simulink model "step3"  (R2021a)
settings: Solver=VariableStepAuto  StartTime=0.0  StopTime=100.0  RelTol=1e-3
settings Model: Creator=konsta  LastModifiedBy=konsta

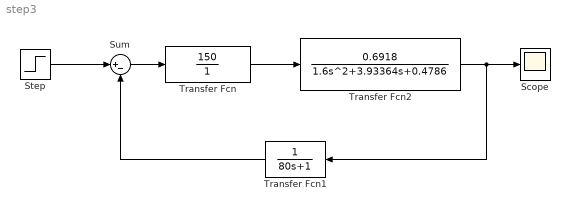
== system step3 ==
  Scope : Scope
  Step : Step  SampleTime=0
  Sum : Sum  Inputs=|+-
  Transfer Fcn : TransferFcn  Numerator=[150]  Denominator=[0 1]
  Transfer Fcn1 : TransferFcn  Denominator=[80 1]
  Transfer Fcn2 : TransferFcn  Numerator=[0.6918]  Denominator=[1.6 3.93364 0.4786]
  wires:
  Transfer Fcn2/1 -> Transfer Fcn1/1, Scope/1
  Transfer Fcn1/1 -> Sum/2
  Sum/1 -> Transfer Fcn/1
  Transfer Fcn/1 -> Transfer Fcn2/1
  Step/1 -> Sum/1
